simulink model "engine_test"  (R2016b)
settings: Solver=VariableStepAuto  StartTime=0.0  StopTime=20  RelTol=1e-3
values from neighbouring files (symbols this model uses):
  A = J*(Omega_phi + Omega)    [IMU.m]
  phase = 6    [calculate_PWM.m]    (also in pwm_test.m)
libraries: powerlib x11
settings Model: Creator=Paweł Tymiński  LastModifiedBy=Paweł Tymiński

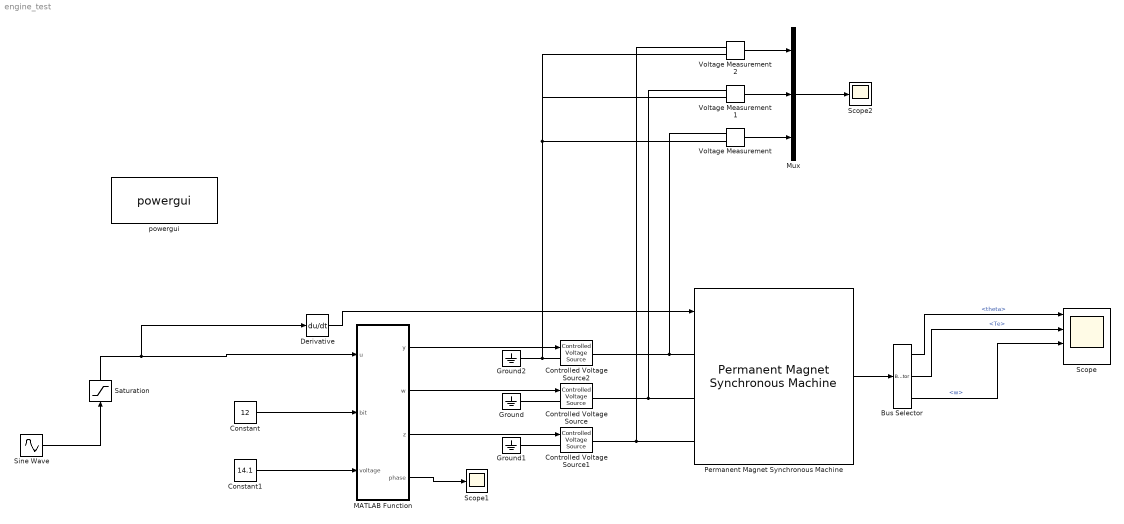
== system engine_test ==
  Bus Selector : BusSelector  OutputSignals=theta,Te,w
  Constant : Constant  Value=12
  Constant1 : Constant  Value=14.1
  Controlled Voltage Source : powerlib/Electrical Sources/Controlled Voltage Source  Initialize=on  Source_Type=DC  Amplitude=12  Phase=0  Frequency=0  Measurements=Voltage
  Controlled Voltage Source1 : powerlib/Electrical Sources/Controlled Voltage Source  Initialize=on  Source_Type=DC  Amplitude=0  Phase=0  Frequency=0  Measurements=Voltage
  Controlled Voltage Source2 : powerlib/Electrical Sources/Controlled Voltage Source  Initialize=on  Source_Type=DC  Amplitude=12  Phase=0  Frequency=0  Measurements=None
  Derivative : Derivative
  Ground : powerlib/Elements/Ground  LConnTagsString=a
  Ground1 : powerlib/Elements/Ground  LConnTagsString=a
  Ground2 : powerlib/Elements/Ground  LConnTagsString=a
  MATLAB Function : MATLAB Function  TreatAsAtomicUnit=on
  Mux : Mux  Inputs=3
  Permanent Magnet Synchronous Machine : powerlib/Machines/Permanent Magnet Synchronous Machine  NbPhases=3  FluxDistribution=Trapezoidal  RotorType=Round  MechanicalLoad=Speed w  PresetModel=No  ShowDetailedParameters=on  MeasurementBus=on  Resistance=0.023  Inductance=0.035  dqInductances=[8.5e-3,8.5e-3]  La=0.00167  MachineConstant=Torque Constant (N.m / A_peak)  Flux=0.044643  VoltageCst=65.4498  TorqueCst=0.625  Flat=120  Mechanical=[0.000621417 4.5 7]  PolePairs=7  InitialConditions=[0,0, 0,0]  InitialConditions5ph=[0 0 0 0 0 0]  TsPowergui=0  TsBlock=0.0003  RefAngle=90 degrees behind phase A axis (modified Park)
  Saturation : Saturate  UpperLimit=360  LowerLimit=-360
  Scope : Scope  NumInputPorts=4
  Scope1 : Scope
  Scope2 : Scope
  Sine Wave : Sin  Amplitude=15  SampleTime=0
  Voltage Measurement : powerlib/Measurements/Voltage Measurement  PhasorSimulation=off  OutputType=Complex  PSBequivalent=0
  Voltage Measurement1 : powerlib/Measurements/Voltage Measurement  PhasorSimulation=off  OutputType=Complex  PSBequivalent=0
  Voltage Measurement2 : powerlib/Measurements/Voltage Measurement  PhasorSimulation=off  OutputType=Complex  PSBequivalent=0
  powergui : powerlib/powergui  Priority=1  SimulationMode=Discrete  SolverType=Tustin/Backward Euler (TBE)  SampleTime=0.01  frequency=60  SPID=off  DisableSnubberDevices=off  DisableRonSwitches=off  DisableVfSwitches=off  SwTol=0  DisplayEquations=off  Interpol=off  ExternalGateDelay=off  methode=off  Ts=10  FunctionMessages=off  echomessages=off  HookPort=off  EnableUseOfTLC=off  x0status=blocks  frequencyindice=0  Pbase=100e6  ErrMax=1e-4  Iterations=50  UnitsV=kV  UnitsW=MW  buscounter=0  RestoreLinks=warning  ResistiveCurrentMeasurement=off  Frange=[0:2:500]  Ylog=off  Xlog=on  ShowGrid=off  save=off  variable=ZData  structure=0  ZoomFFT=off  StartTime=0.0  cycles=1  DisplayStyle=1  fundamental=60  FreqAxis=off  MaxFrequency=1000  frequencyindicesteady=1  RmsSteady=1  display=off
  wires:
  Constant1/1 -> MATLAB Function/3(voltage)
  MATLAB Function/4(phase) -> Scope1/1
  Constant/1 -> MATLAB Function/2(bit)
  Voltage Measurement/1 -> Mux/3
  Voltage Measurement2/1 -> Mux/1
  Voltage Measurement1/1 -> Mux/2
  Permanent Magnet Synchronous Machine/1 -> Bus Selector/1
  Sine Wave/1 -> Saturation/1
  MATLAB Function/1(y) -> Controlled Voltage Source2/1
  MATLAB Function/2(w) -> Controlled Voltage Source/1
  MATLAB Function/3(z) -> Controlled Voltage Source1/1
  Mux/1 -> Scope2/1
  Saturation/1 -> Derivative/1, MATLAB Function/1(u)
  Bus Selector/1 -> Scope/1  "<theta>"
  Bus Selector/2 -> Scope/2  "<Te>"
  Derivative/1 -> Permanent Magnet Synchronous Machine/1
  Bus Selector/3 -> Scope/3  "<w>"
  connections:
  Permanent Magnet Synchronous Machine/LConn1 -- Voltage Measurement/LConn1 -- Controlled Voltage Source2/RConn1
  Ground/LConn1 -- Controlled Voltage Source/LConn1
  Ground1/LConn1 -- Controlled Voltage Source1/LConn1
  Permanent Magnet Synchronous Machine/LConn2 -- Voltage Measurement1/LConn1 -- Controlled Voltage Source/RConn1
  Permanent Magnet Synchronous Machine/LConn3 -- Voltage Measurement2/LConn1 -- Controlled Voltage Source1/RConn1
  Ground2/LConn1 -- Voltage Measurement/LConn2 -- Voltage Measurement1/LConn2 -- Voltage Measurement2/LConn2 -- Controlled Voltage Source2/LConn1

== matlab function engine_test/MATLAB Function ==
  data: u input; y output; bit input; voltage input; w output; z output; phase output

function[y,w,z,phase] = calculate_PWM(u,bit,voltage)
%konwersja kąta na wartości sygnału PWM do sterowania silnikiem BLDC
nop = 14;
phase=1;
PWM=0;
resolution = 2^bit; %rozdzielczość bitowa generowanego sygnału
    y=voltage;
    w=voltage;
    z=0;
%kalkulacja wartości PWM na poszczególne fazy

%konwersja kąta na wejściu na radiany
theta_error = deg2rad(u);

%konwersja kąta mechanicznego na elektryczny (poślizg silnika)
theta_e = (theta_error*nop)/2;
%ograniczenie wartości kąta do wartości z zakresu 0-2 pi
theta_e = mod(theta_e,(2*pi));
if(theta_e < 0)
        theta_e = theta_e + (2*pi);
end

  if  theta_e <= 2/6*pi && theta_e>0
    PWM =round(resolution*(tan(theta_e)) /  (sin(2/3*pi)-cos(2/3*pi)*tan(theta_e)));
    phase=1;
elseif theta_e <= 4/6*pi && theta_e>2/6*pi
    PWM =round(resolution*-((tan(theta_e)*cos(2/3*pi)-sin(2/3*pi))/tan(theta_e)));
    phase=2;
elseif theta_e <= 6/6*pi && theta_e>4/6*pi
    PWM =round(resolution*(tan(theta_e)*cos(2/3*pi)-sin(2/3*pi)/sin(4/3*pi) -cos(4/3*pi)*tan(theta_e)));
    phase=3;
elseif theta_e <= 8/6*pi && theta_e>6/6*pi
    PWM =round(resolution*(tan(theta_e)*cos(4/3*pi)-sin(4/3*pi)/sin(2/3*pi) -cos(2/3*pi)*tan(theta_e)));
    phase=4;   
elseif theta_e <= 10/6*pi && theta_e>8/6*pi
    PWM =round(resolution*(sin(4/3*pi) - tan(theta_e)*cos(4/3*pi))/tan(theta_e));
    phase=5;
elseif theta_e <= 12/6*pi && theta_e>10/6*pi
    PWM =round(resolution*(tan(theta_e))/(sin(4/3*pi)-cos(4/3*pi)*tan(theta_e)));
    phase=6;
 end


if(phase==1)
    y=voltage;
    w=(voltage/resolution)*PWM;
    z=0;
elseif(phase==2)
    y=(voltage/resolution)*PWM;
    w=voltage;
    z=0;
elseif(phase==3)
    y=0;
    w=voltage;
    z=(voltage/resolution)*PWM;
elseif(phase==4)
    y=0;
    w=(voltage/resolution)*PWM;
    z=voltage;
elseif(phase==5)
    y=(voltage/resolution)*PWM;
    w=0;
    z=voltage;
else
    y=voltage;
    w=0;
    z=(voltage/resolution)*PWM;
end
end
